simulink model "TRAS_controller_2013"  (R2013a)
settings: Solver=ode3  SolverMode=SingleTasking  StartTime=0.0  StopTime=stop_time  FixedStep=sampling_time  RelTol=1e-3
values from neighbouring files (symbols this model uses):
  A = 0.0552    [momentsOfInertia.m]
  B = 0.0599    [momentsOfInertia.m]
  C = 0.0084    [momentsOfInertia.m]
  D = (mmr + mms + mm / 3) * lm^2 + (mtr + mts + mt / 3) * lt^2    (= 0.0224143186667)    [momentsOfInertia.m]
  derivative_pole_tc = 2 * sampling_time    (= 0.02)    [TRAS_closed_loop.m]
  F = mms * rms^2 + mts * rts^2    (= 0.002355075)    [momentsOfInertia.m]
  Fh_force_grid = polyval(Fh, Fh_omega_grid)    [thrustForcesDependencies.m]
  Fh_omega_grid = linspace(-4000, 4000, 1e4)    [thrustForcesDependencies.m]
  Fv_force_grid = polyval(Fv, Fv_omega_grid)    [thrustForcesDependencies.m]
  Fv_omega_grid = linspace(-4000, 4000, 1e4)    [thrustForcesDependencies.m]
  g = 9.81    [TRAS_closed_loop.m]    (also in TRAS_controller.m; TRAS_process.m)
  Jv = D + E + F    (= 0.0253918936667)    [momentsOfInertia.m]
  kd = 2 * zeta * wn + pole    (= 8.88888888889)    [TRAS_closed_loop.m]    (also in TRAS_controller.m = 4)
  ki = pole * wn^2    (= 7.80368846212)    [TRAS_closed_loop.m]
  ki_inner = wn_inner^2    (= 23.7953599048)    [TRAS_closed_loop.m]
  kp = wn^2 + 2 * zeta * wn * pole    (= 15.890260631)    [TRAS_closed_loop.m]    (also in TRAS_controller.m = 4)
  kp_inner = 2 * zeta_inner * wn_inner    (= 8)    [TRAS_closed_loop.m]
  L = (mmr + mms + mm / 4) * lm^2 + (mtr + mts + mt / 4) * lt^2 - mcb * lcb^2 - mb / 4 * lb^2    (= 0.021593306)    [momentsOfInertia.m]
  lm = 0.202    [momentsOfInertia.m]
  lt = 0.216    [momentsOfInertia.m]
settings Model: CovMetricSettings=dwe  CovHtmlReporting=off  covSaveCumulativeToWorkspaceVar=off  CovSaveSingleToWorkspaceVar=off  CovExternalEMLEnable=on  Creator=Codrin  LastModifiedBy=Codrin
settings DataIOCC: LimitDataPoints=off  SaveFormat=StructureWithTime  ReturnWorkspaceOutputs=on
settings DebuggingCC: UnderspecifiedInitializationDetection=Simplified  MergeDetectMultiDrivingBlocksExec=error  SolverPrmCheckMsg=none  UnconnectedInputMsg=none  UnconnectedOutputMsg=none  UnconnectedLineMsg=none  FrameProcessingCompatibilityMsg=error  StateNameClashWarn=none  SFUnexpectedBacktrackingDiag=error  SFNoUnconditionalDefaultTransitionDiag=error
settings HardwareCC: ProdBitPerPointer=64  ProdLargestAtomicFloat=Float  ProdIntDivRoundTo=Zero  ProdEndianess=LittleEndian  ProdHWDeviceType=Specified
settings ModelReferenceCC: PropagateSignalLabelsOutOfModel=on
settings SFSimCC: SimUseLocalCustomCode=on
settings RTWCC: RTWUseLocalCustomCode=on
settings GRTTargetCC: CodeReplacementLibrary=C99 (ISO)

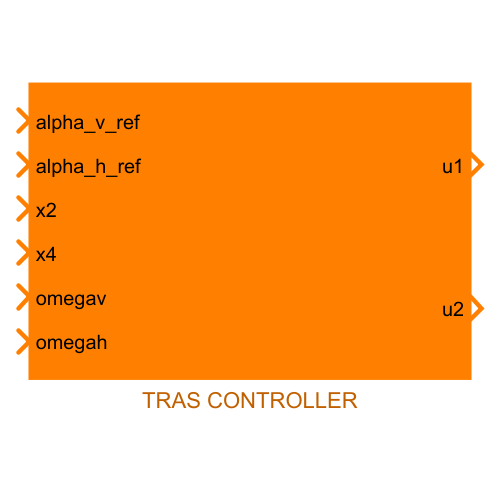
[thumbnail: Simulink's stored preview of the top-level diagram]
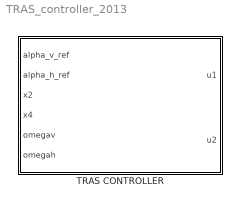
== system TRAS_controller_2013 ==
  TRAS CONTROLLER : Subsystem

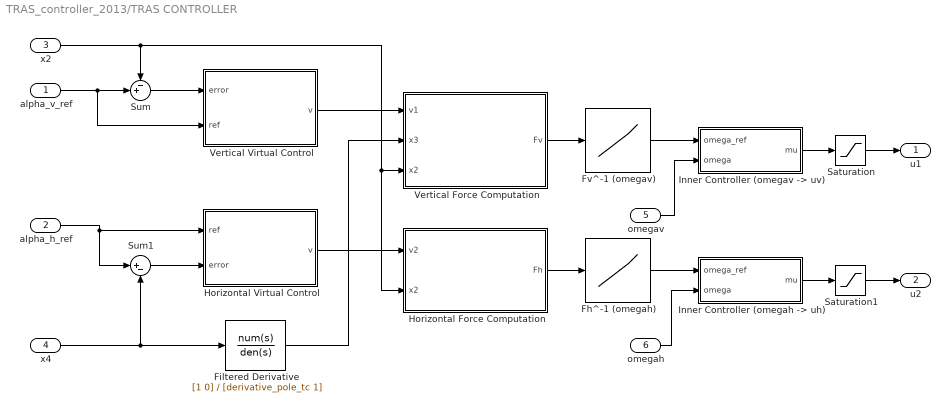
== system TRAS_controller_2013/TRAS CONTROLLER ==
  alpha_v_ref : Inport
  alpha_h_ref : Inport  Port=2
  x2 : Inport  Port=3
  x4 : Inport  Port=4
  omegav : Inport  Port=5
  omegah : Inport  Port=6
  Fh^-1 (omegah) : Lookup_n-D  NumberOfTableDimensions=1  BreakpointsForDimension1=Fh_force_grid  Table=Fh_omega_grid  ExtrapMethod=Clip  RndMeth=Simplest  InputSameDT=on
  Filtered Derivative : TransferFcn  Numerator=[1 0]  Denominator=[derivative_pole_tc 1]
  Fv^-1 (omegav) : Lookup_n-D  NumberOfTableDimensions=1  BreakpointsForDimension1=Fv_force_grid  Table=Fv_omega_grid  ExtrapMethod=Clip  RndMeth=Simplest  InputSameDT=on
  Horizontal Force Computation : MATLAB Function  TreatAsAtomicUnit=on
      settings: PermitHierarchicalResolution=ParametersOnly
  Horizontal Virtual Control : Subsystem
  "Inner Controller (omegah -> uh)" : Subsystem
  "Inner Controller (omegav -> uv)" : Subsystem
  Saturation : Saturate  UpperLimit=0.98  LowerLimit=-0.98
  Saturation1 : Saturate  UpperLimit=0.98  LowerLimit=-0.98
  Sum : Sum  Inputs=-+|
  Sum1 : Sum  Inputs=|+-
  Vertical Force Computation : MATLAB Function  TreatAsAtomicUnit=on
      settings: PermitHierarchicalResolution=ParametersOnly
  Vertical Virtual Control : Subsystem
  u1 : Outport
  u2 : Outport  Port=2
  wires:
  Filtered Derivative/1 -> Vertical Force Computation/2(x3)
  Vertical Virtual Control/1(v) -> Vertical Force Computation/1(v1)
  x2/1 -> Horizontal Force Computation/2(x2), Vertical Force Computation/3(x2), Sum/1
  Horizontal Virtual Control/1(v) -> Horizontal Force Computation/1(v2)
  x4/1 -> Sum1/2, Filtered Derivative/1
  alpha_v_ref/1 -> Vertical Virtual Control/2(ref), Sum/2
  alpha_h_ref/1 -> Horizontal Virtual Control/1(ref), Sum1/1
  Sum1/1 -> Horizontal Virtual Control/2(error)
  "Inner Controller (omegav -> uv)"/1(mu) -> Saturation/1
  omegav/1 -> "Inner Controller (omegav -> uv)"/2(omega)
  "Inner Controller (omegah -> uh)"/1(mu) -> Saturation1/1
  omegah/1 -> "Inner Controller (omegah -> uh)"/2(omega)
  Sum/1 -> Vertical Virtual Control/1(error)
  Vertical Force Computation/1(Fv) -> Fv^-1 (omegav)/1
  Horizontal Force Computation/1(Fh) -> Fh^-1 (omegah)/1
  Fh^-1 (omegah)/1 -> "Inner Controller (omegah -> uh)"/1(omega_ref)
  Fv^-1 (omegav)/1 -> "Inner Controller (omegav -> uv)"/1(omega_ref)
  Saturation1/1 -> u2/1
  Saturation/1 -> u1/1

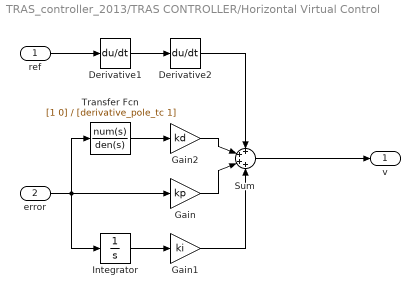
== system TRAS_controller_2013/TRAS CONTROLLER/Horizontal Virtual Control ==
  ref : Inport
  error : Inport  Port=2
  Derivative1 : Derivative
  Derivative2 : Derivative
  Gain : Gain  Gain=kp
  Gain1 : Gain  Gain=ki
  Gain2 : Gain  Gain=kd
  Integrator : Integrator
  Sum : Sum  Inputs=++++
  Transfer Fcn : TransferFcn  Numerator=[1 0]  Denominator=[derivative_pole_tc 1]
  v : Outport
  wires:
  Sum/1 -> v/1
  Gain1/1 -> Sum/4
  Gain/1 -> Sum/3
  Gain2/1 -> Sum/2
  Derivative2/1 -> Sum/1
  Transfer Fcn/1 -> Gain2/1
  error/1 -> Transfer Fcn/1, Gain/1, Integrator/1
  Derivative1/1 -> Derivative2/1
  ref/1 -> Derivative1/1
  Integrator/1 -> Gain1/1

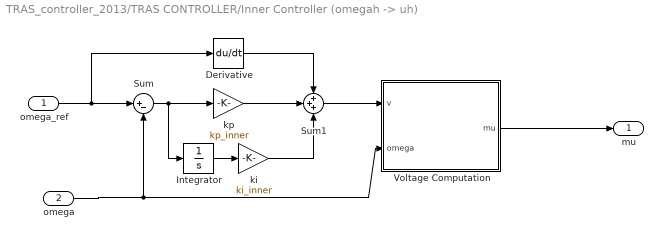
== system TRAS_controller_2013/TRAS CONTROLLER/Inner Controller (omegah -> uh) ==
  omega_ref : Inport
  omega : Inport  Port=2
  Derivative : Derivative
  Integrator : Integrator
  Sum : Sum  Inputs=|+-
  Sum1 : Sum  Inputs=+++
  Voltage Computation : MATLAB Function  TreatAsAtomicUnit=on
      settings: PermitHierarchicalResolution=ParametersOnly
  ki : Gain  Gain=ki_inner
  kp : Gain  Gain=kp_inner
  mu : Outport
  wires:
  ki/1 -> Sum1/3
  Integrator/1 -> ki/1
  Voltage Computation/1(mu) -> mu/1
  Sum1/1 -> Voltage Computation/1(v)
  Derivative/1 -> Sum1/1
  kp/1 -> Sum1/2
  Sum/1 -> kp/1, Integrator/1
  omega_ref/1 -> Sum/1, Derivative/1
  omega/1 -> Voltage Computation/2(omega), Sum/2

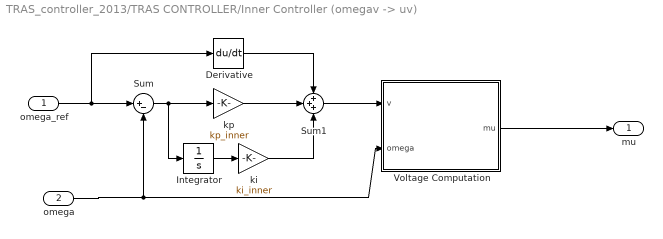
== system TRAS_controller_2013/TRAS CONTROLLER/Inner Controller (omegav -> uv) ==
  omega_ref : Inport
  omega : Inport  Port=2
  Derivative : Derivative
  Integrator : Integrator
  Sum : Sum  Inputs=|+-
  Sum1 : Sum  Inputs=+++
  Voltage Computation : MATLAB Function  TreatAsAtomicUnit=on
      settings: PermitHierarchicalResolution=ParametersOnly
  ki : Gain  Gain=ki_inner
  kp : Gain  Gain=kp_inner
  mu : Outport
  wires:
  omega/1 -> Sum/2, Voltage Computation/2(omega)
  omega_ref/1 -> Derivative/1, Sum/1
  Sum/1 -> Integrator/1, kp/1
  kp/1 -> Sum1/2
  Derivative/1 -> Sum1/1
  Sum1/1 -> Voltage Computation/1(v)
  Voltage Computation/1(mu) -> mu/1
  Integrator/1 -> ki/1
  ki/1 -> Sum1/3

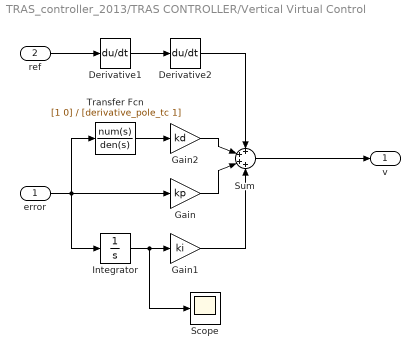
== system TRAS_controller_2013/TRAS CONTROLLER/Vertical Virtual Control ==
  error : Inport
  ref : Inport  Port=2
  Derivative1 : Derivative
  Derivative2 : Derivative
  Gain : Gain  Gain=kp
  Gain1 : Gain  Gain=ki
  Gain2 : Gain  Gain=kd
  Integrator : Integrator  LimitOutput=on  UpperSaturationLimit=0.2  LowerSaturationLimit=-0.2
  Scope : Scope
      settings: TimeRange=auto  MaxDataPoints=5000  SaveToWorkspace=off  SaveName=ScopeData3  YMin=-0.02037  YMax=0.03808  SampleTime=-1
  Sum : Sum  Inputs=++++
  Transfer Fcn : TransferFcn  Numerator=[1 0]  Denominator=[derivative_pole_tc 1]
  v : Outport
  wires:
  Integrator/1 -> Scope/1, Gain1/1
  ref/1 -> Derivative1/1
  Derivative1/1 -> Derivative2/1
  error/1 -> Transfer Fcn/1, Integrator/1, Gain/1
  Transfer Fcn/1 -> Gain2/1
  Derivative2/1 -> Sum/1
  Gain2/1 -> Sum/2
  Gain/1 -> Sum/3
  Gain1/1 -> Sum/4
  Sum/1 -> v/1

== matlab function TRAS_controller_2013/TRAS CONTROLLER/Vertical Force Computation ==
  data: Fv output; v1 input; x3 input; x2 input; Jv parameter; L parameter; g parameter; A parameter; B parameter; C parameter; lm parameter
function Fv = verticalForceComputation(v1, x3, x2, Jv, L, g, A, B, C, lm)

Fv = 1 / lm * (v1 * Jv + x3^2 / 2 * L * sin(2 * x2) - g * ((A-B)*cos(x2) - C*sin(x2)));

== matlab function TRAS_controller_2013/TRAS CONTROLLER/Horizontal Force Computation ==
  data: v2 input; Fh output; x2 input; lt parameter; D parameter; E parameter; F parameter
function Fh = horizontalForceComputation(v2, x2, lt, D, E, F)

Fh = v2 / (lt * cos(x2)) * (D * cos(x2)^2 + E * sin(x2)^2 + F);

== matlab function TRAS_controller_2013/TRAS CONTROLLER/Inner Controller (omegav -> uv)/Voltage Computation ==
  data: v input; mu output; omega input; Thetav parameter
function mu = PWMComputation(v, omega, Thetav)

%case1 : suppose mu >= 0
mu = (v + Thetav(3) * omega + omega * abs(omega) * Thetav(4)) / (Thetav(1) - Thetav(2));

if(mu < 0) %case 2: mu < 0
    mu = (v + Thetav(3) * omega + omega * abs(omega) * Thetav(4)) / (Thetav(1) + Thetav(2));
end

== matlab function TRAS_controller_2013/TRAS CONTROLLER/Inner Controller (omegah -> uh)/Voltage Computation ==
  data: v input; mu output; omega input; Thetav parameter
function mu = PWMComputation(v, omega, Thetav)

%case1 : suppose mu >= 0
mu = (v + Thetav(3) * omega + omega * abs(omega) * Thetav(4)) / (Thetav(1) - Thetav(2));

if(mu < 0) %case 2: mu < 0
    mu = (v + Thetav(3) * omega + omega * abs(omega) * Thetav(4)) / (Thetav(1) + Thetav(2));
end
